simulink model "Sistema_Seguimiento_Final_2021"  (R2016a)
settings: Solver=VariableStepAuto  StartTime=0.0  StopTime=3  RelTol=1e-3
values from neighbouring files (symbols this model uses):
  K = acker(A, B ,PLC)    [Final_2017_Ejercicio_3.m]    (also in Final_2018_Ejercicio_1.m; Final_2018_Ejercicio_2.m = 10; Final_2019_Ejercicio_3.m = acker(Ahat, Bhat ,PLC2); Final_2020.m = acker(Ahat, Bhat ,PLC))
libraries: simulink x1
settings Model: Creator=Abel  LastModifiedBy=Abel

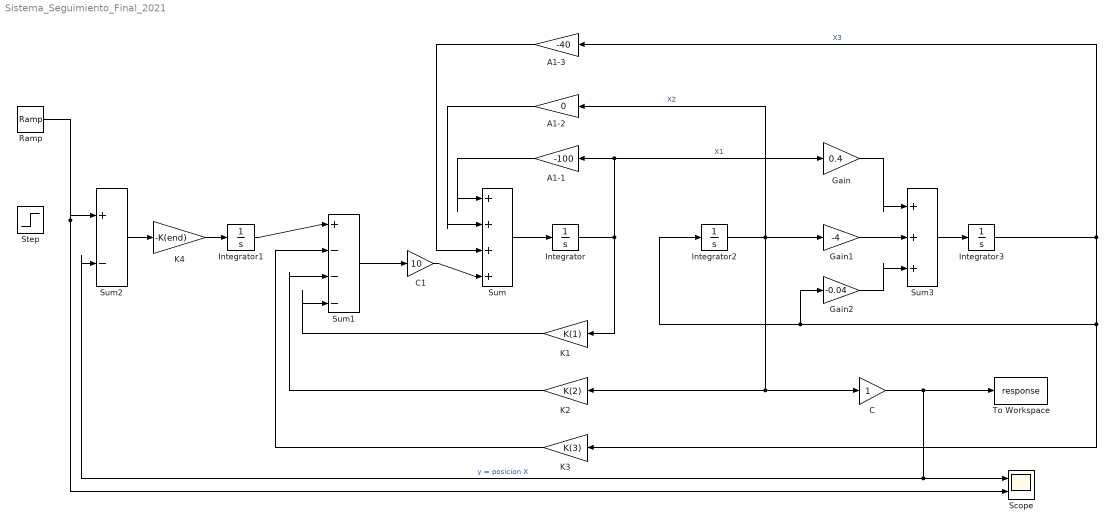
== system Sistema_Seguimiento_Final_2021 ==
  A1-1 : Gain  Gain=-100
  A1-2 : Gain  Gain=0
  A1-3 : Gain  Gain=-40
  C : Gain
  C1 : Gain  Gain=10
  Gain : Gain  Gain=0.4
  Gain1 : Gain  Gain=-4
  Gain2 : Gain  Gain=-0.04
  Integrator{,1..3} (4 alike) : Integrator
  K1 : Gain  Gain=K(1)
  K2 : Gain  Gain=K(2)
  K3 : Gain  Gain=K(3)
  K4 : Gain  Gain=-K(end)
  Ramp : simulink/Sources/Ramp  slope=1  start=0  X0=0
  Scope : Scope  NumInputPorts=2
  Step : Step  Time=0  SampleTime=0
  Sum : Sum  Inputs=|+|+|+|+|
  Sum1 : Sum  Inputs=|+|-|-|-|
  Sum2 : Sum  Inputs=|+|-|
  Sum3 : Sum  Inputs=|+|+|+|
  To Workspace : ToWorkspace  VariableName=response  SaveFormat=Timeseries  SampleTime=-1
      settings: Save2DSignal=2-D array (concatenate along first dimension)
  wires:
  Integrator/1 -> K1/1, Gain/1, A1-1/1  "X1"
  Sum/1 -> Integrator/1
  A1-1/1 -> Sum/1
  A1-2/1 -> Sum/2
  Integrator2/1 -> Gain1/1, K2/1, C/1, A1-2/1  "X2"
  Sum2/1 -> K4/1
  Integrator3/1 -> Integrator2/1, Gain2/1, K3/1, A1-3/1  "X3"
  C/1 -> Sum2/2, Scope/1, To Workspace/1  "y = posicion X"
  A1-3/1 -> Sum/3
  K1/1 -> Sum1/4
  K2/1 -> Sum1/3
  K3/1 -> Sum1/2
  K4/1 -> Integrator1/1
  Integrator1/1 -> Sum1/1
  Sum3/1 -> Integrator3/1
  Gain/1 -> Sum3/1
  Gain1/1 -> Sum3/2
  Gain2/1 -> Sum3/3
  C1/1 -> Sum/4
  Sum1/1 -> C1/1
  Ramp/1 -> Scope/2, Sum2/1
